simulink model "ccu_form"  (R2019b)
settings: Solver=FixedStepDiscrete  StartTime=0.0  StopTime=10.0  FixedStep=0.0005  RelTol=1e-3
undefined symbols (not defined in the file): CubeAndKeil, DiscIntNeverNeededParam, Ggg2
libraries: simulink x6, GPIO_Lib x5, ADC_Lib x2, TIMERS_Lib x2, USART_Lib x2, STM32_Config_Lib x1
settings Model: Creator=Guest  LastModifiedBy=Dmitry
settings OptimizationCC: DefaultParameterBehavior=Inlined  OptimizeBlockIOStorage=off  BufferReuse=off  GlobalBufferReuse=off  ExpressionFolding=off  EnableMemcpy=off  PassReuseOutputArgsAs=Individual arguments  LocalBlockOutputs=off  ZeroExternalMemoryAtStartup=off  ZeroInternalMemoryAtStartup=off  OptimizeDataStoreBuffers=off  BusAssignmentInplaceUpdate=off  OptimizationLevel=level0  OptimizationCustomize=off  EfficientTunableParamExpr=on
settings DebuggingCC: MultiTaskDSMMsg=none  ParameterOverflowMsg=none  ParameterTunabilityLossMsg=error
settings HardwareCC: ProdBitPerPointer=32  ProdBitPerSizeT=32  ProdBitPerPtrDiffT=32  ProdLargestAtomicInteger=Long  ProdWordSize=32  ProdHWDeviceType=STM32CortexM
settings SFSimCC: MATLABDynamicMemAlloc=off
settings RTWCC: Description=stm32 (Embedded Target)  SystemTargetFile=stm32.tlc  TemplateMakefile=stm32.tmf  GenerateReport=on  IncludeHyperlinkInReport=on  GenerateTraceInfo=on  GenerateTraceReport=on  GenerateTraceReportSl=on  GenerateTraceReportSf=on  GenerateTraceReportEml=on
settings CodeAppCC: ForceParamTrailComments=on  IgnoreCustomStorageClasses=off  MaxIdLength=64  OperatorAnnotations=on  SimulinkDataObjDesc=on  SFDataObjDesc=on  CustomSymbolStrType=$N$R$M
settings STFCustomTargetCC: TargetLangStandard=C99 (ISO)  CodeReplacementLibrary=ARM CMSIS SIN COS  MultiwordLength=256  ParMdlRefBuildCompliant=on  IncludeMdlTerminateFcn=off  CombineOutputUpdateFcns=on  ERTCustomFileBanners=on  SupportContinuousTime=off  SupportNonInlinedSFcns=off  RemoveResetFunc=on  MATLABClassNameForMDSCustomization=Simulink.SoftwareTarget.ERTCustomization  SystemTargetFile=stm32.tlc
settings ERTTargetCC: TargetLangStandard=C99 (ISO)  CodeReplacementLibrary=ARM CMSIS SIN COS  CompOptLevelCompliant=off  ConcurrentExecutionCompliant=off  IncludeMdlTerminateFcn=off  ModelStepFunctionPrototypeControlCompliant=off  CPPClassGenCompliant=off  UseToolchainInfoCompliant=off  ExtModeStaticAllocSize=256  ExtModeMexFile=ext_serial_win32_comm  ExtModeMexArgs=0,1,115200,10  InlinedParameterPlacement=NonHierarchical  ERTSrcFileBannerTemplate=sourceFileTemplate.cgt  ERTHdrFileBannerTemplate=sourceFileTemplate.cgt  ERTDataSrcFileTemplate=sourceFileTemplate.cgt  ERTDataHdrFileTemplate=sourceFileTemplate.cgt  ERTCustomFileTemplate=customRoutineProcess.tlc

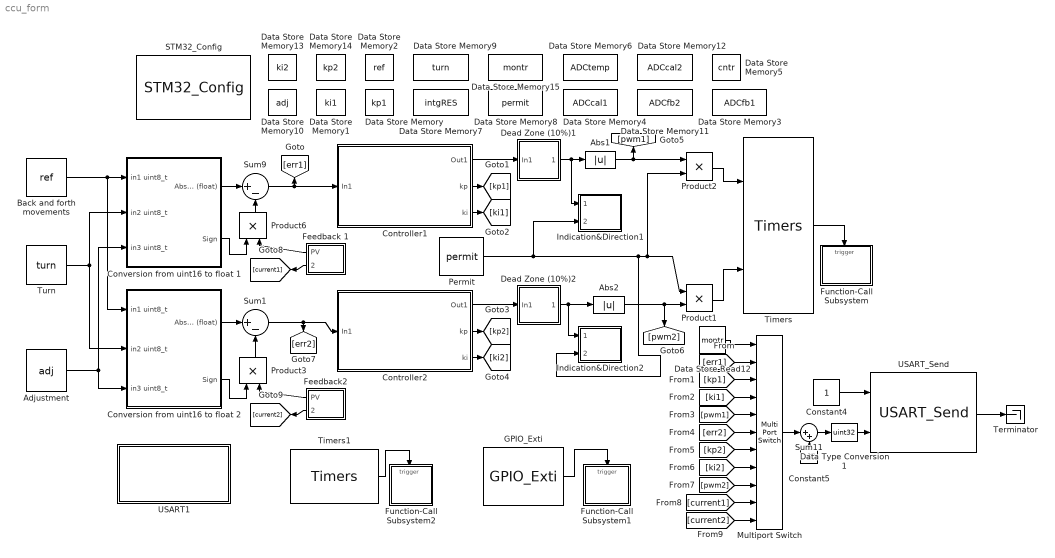
== system ccu_form ==
  Abs1 : Abs
  Abs2 : Abs
  Adjustment : DataStoreRead  DataStoreName=adj  DataStoreElements=adj
      mask Display: image('E:\diplom\matlab\handle.png','center')
  Back and forth movements : DataStoreRead  DataStoreName=ref  DataStoreElements=ref
      mask Display: image('E:\diplom\matlab\joystick_fb.png','center')
  Constant4 : Constant
  Constant5 : Constant  Value=100  OutDataTypeStr=uint8
  Controller1 : Subsystem
      mask Display: image('E:\diplom\matlab\pi.png','center')
  Controller2 : Subsystem
      mask Display: image('E:\diplom\matlab\pi.png','center')
  Conversion from uint16 to float 1 : Subsystem
  Conversion from uint16 to float 2 : Subsystem
  Data Store Memory : DataStoreMemory  DataStoreName=kp1  ReadBeforeWriteMsg=warning  WriteAfterWriteMsg=warning  WriteAfterReadMsg=warning  ShowAdditionalParam=off  OutDataTypeStr=uint8
  Data Store Memory1 : DataStoreMemory  DataStoreName=ki1  ReadBeforeWriteMsg=warning  WriteAfterWriteMsg=warning  WriteAfterReadMsg=warning  ShowAdditionalParam=off  OutDataTypeStr=uint8
  Data Store Memory10 : DataStoreMemory  DataStoreName=adj  ReadBeforeWriteMsg=warning  WriteAfterWriteMsg=warning  WriteAfterReadMsg=warning  ShowAdditionalParam=off  OutDataTypeStr=uint8
  Data Store Memory11 : DataStoreMemory  DataStoreName=ADCfb2  ReadBeforeWriteMsg=warning  WriteAfterWriteMsg=warning  WriteAfterReadMsg=warning  ShowAdditionalParam=off  OutDataTypeStr=uint16
  Data Store Memory12 : DataStoreMemory  DataStoreName=ADCcal2  ReadBeforeWriteMsg=warning  WriteAfterWriteMsg=warning  WriteAfterReadMsg=warning  ShowAdditionalParam=off  OutDataTypeStr=uint16
  Data Store Memory13 : DataStoreMemory  DataStoreName=ki2  ReadBeforeWriteMsg=warning  WriteAfterWriteMsg=warning  WriteAfterReadMsg=warning  ShowAdditionalParam=off  OutDataTypeStr=uint8
  Data Store Memory14 : DataStoreMemory  DataStoreName=kp2  ReadBeforeWriteMsg=warning  WriteAfterWriteMsg=warning  WriteAfterReadMsg=warning  ShowAdditionalParam=off  OutDataTypeStr=uint8
  Data Store Memory15 : DataStoreMemory  DataStoreName=montr  ReadBeforeWriteMsg=warning  WriteAfterWriteMsg=warning  WriteAfterReadMsg=warning  ShowAdditionalParam=off  OutDataTypeStr=uint8
  Data Store Memory2 : DataStoreMemory  DataStoreName=ref  ReadBeforeWriteMsg=warning  WriteAfterWriteMsg=warning  WriteAfterReadMsg=warning  ShowAdditionalParam=off  OutDataTypeStr=uint8
  Data Store Memory3 : DataStoreMemory  DataStoreName=ADCfb1  ReadBeforeWriteMsg=warning  WriteAfterWriteMsg=warning  WriteAfterReadMsg=warning  ShowAdditionalParam=off  OutDataTypeStr=uint16
  Data Store Memory4 : DataStoreMemory  DataStoreName=ADCcal1  ReadBeforeWriteMsg=warning  WriteAfterWriteMsg=warning  WriteAfterReadMsg=warning  ShowAdditionalParam=off  OutDataTypeStr=uint16
  Data Store Memory5 : DataStoreMemory  DataStoreName=cntr  ReadBeforeWriteMsg=warning  WriteAfterWriteMsg=warning  WriteAfterReadMsg=warning  ShowAdditionalParam=off  OutDataTypeStr=uint16
  Data Store Memory6 : DataStoreMemory  DataStoreName=ADCtemp  ReadBeforeWriteMsg=warning  WriteAfterWriteMsg=warning  WriteAfterReadMsg=warning  ShowAdditionalParam=off  OutDataTypeStr=uint32
  Data Store Memory7 : DataStoreMemory  DataStoreName=intgRES  ReadBeforeWriteMsg=warning  WriteAfterWriteMsg=warning  WriteAfterReadMsg=warning  ShowAdditionalParam=off  OutDataTypeStr=uint8
  Data Store Memory8 : DataStoreMemory  DataStoreName=permit  ReadBeforeWriteMsg=warning  WriteAfterWriteMsg=warning  WriteAfterReadMsg=warning  ShowAdditionalParam=off  OutDataTypeStr=uint8
  Data Store Memory9 : DataStoreMemory  DataStoreName=turn  ReadBeforeWriteMsg=warning  WriteAfterWriteMsg=warning  WriteAfterReadMsg=warning  ShowAdditionalParam=off  OutDataTypeStr=uint8
  Data Store Read12 : DataStoreRead  DataStoreName=montr  DataStoreElements=montr
  Data Type Conversion1 : DataTypeConversion  OutDataTypeStr=uint32
  Dead Zone (10%)1 : Subsystem
      mask Display:
      | plot([0.01 1 1.01 3 3.01 4.01],[-1.00001 -0.5 0.00001 0 0.5 1.01])
      | plot([0.0001 1.0001 1.0001 3.0001 3.0001 4.00001],[-1.0001 -0.50001 0.0001 0.0001 0.5001 1.0001])
      | plot([0.0002 1.0002 1.001 3.001 3.001 4.0001],[-1.0005 -0.50005 0.0005 0.0005 0.5005 1.0005])
      | plot([2 2],[-1 1])
      | plot([0 4],[0 0])
  Dead Zone (10%)2 : Subsystem
      mask Display:
      | plot([0.01 1 1.01 3 3.01 4.01],[-1.00001 -0.5 0.00001 0 0.5 1.01])
      | plot([0.0001 1.0001 1.0001 3.0001 3.0001 4.00001],[-1.0001 -0.50001 0.0001 0.0001 0.5001 1.0001])
      | plot([0.0002 1.0002 1.001 3.001 3.001 4.0001],[-1.0005 -0.50005 0.0005 0.0005 0.5005 1.0005])
      | plot([2 2],[-1 1])
      | plot([0 4],[0 0])
  Feedback 1 : Subsystem
  Feedback2 : Subsystem
  Function-Call Subsystem : Subsystem  TreatAsAtomicUnit=on
  Function-Call Subsystem1 : Subsystem  TreatAsAtomicUnit=on
  Function-Call Subsystem2 : Subsystem  TreatAsAtomicUnit=on
  GPIO_Exti : GPIO_Lib/GPIO_Exti  Port_name=GPIOA  Pin_0=off  Pin_1=off  Pin_2=off  Pin_3=off  Pin_4=on  Pin_5=off  Pin_6=off  Pin_7=off  Pin_8=off  Pin_9=off  Pin_10=off  Pin_11=off  Pin_12=off  Pin_13=off  Pin_14=off  Pin_15=off  PinList=GPIOA4
      settings: SourceProductName=Target Support Package - STM32 Adapter
  Indication&Direction1 : Subsystem
  Indication&Direction2 : Subsystem
  Multiport Switch : MultiPortSwitch  Inputs=10  OutDataTypeStr=uint8
  Permit : DataStoreRead  DataStoreName=permit  DataStoreElements=permit
      mask Display: image('E:\diplom\matlab\switch.png','center')
  Product1 : Product
  Product2 : Product
  Product3 : Product  OutDataTypeStr=double
  Product6 : Product  OutDataTypeStr=double
  STM32_Config : STM32_Config_Lib/STM32_Config  Priority=0  Project_Path=.\..\CubeAndKeil\Ggg2\  Config_File=Ggg2.ioc  MCU_Name=STM32F401CCUx
      settings: SourceProductName=Target Support Package - STM32 Adapter
  Sum1 : Sum  Inputs=|+-  AccumDataTypeStr=double  OutDataTypeStr=double
  Sum11 : Sum  Inputs=|++  AccumDataTypeStr=double  OutDataTypeStr=double
  Sum9 : Sum  Inputs=|+-  AccumDataTypeStr=double  OutDataTypeStr=double
  Terminator : Terminator
  Timers : TIMERS_Lib/Timers  currentTIM=TIM1  TIM_Name=TIM1  sysUsingTimer=off  TIM_APBClock=84000000  TIM_Set_Clk=off  TIM_Prescaler=0  TIM_Clock=84000000.00  Variable_frequency=off  TIM_Set_OutFreq=off  TIM_ARR=4201  Output_frequency=19995.24  Repetition_counter=0  TIM_Mode=Center_Aligned_3  TIM_DMA=none  TIM_IRQ=on  TIM_IRQ_ONLY=off  TIM_UP=off  TIM_TRG=off  TIM_COM=off  TIM_BRK=off  NbTIM=2  CH1_enable=on  CH1N_enable=on  CH1_type=Output_PWM  CH1_DMA=off  CH1_int=off  CH1_edge=Rising  CH1_div=1  CH1_variable_duty=on  CH1_set_pulse=off  CH1_output_duty=49.99  CH1_pulse=2100  CH2_enable=on  CH2N_enable=off  CH2_type=Output_Comp  CH2_DMA=off  CH2_int=on  CH2_edge=Rising  CH2_div=1  CH2_variable_duty=off  CH2_set_pulse=off  CH2_output_duty=0.00  CH2_pulse=0  CH3_enable=on  CH3N_enable=off  CH3_type=Output_PWM  CH3_DMA=off  CH3_int=off  CH3_edge=Rising  CH3_div=1  CH3_variable_duty=on  CH3_set_pulse=off  CH3_output_duty=49.99  CH3_pulse=2100  CH4_enable=off  CH4N_enable=off  CH4_type=Unknown  CH4_DMA=off  CH4_int=off  CH4_edge=Rising  CH4_div=1  CH4_variable_duty=off  CH4_set_pulse=off  CH4_output_duty=0.00  CH4_pulse=0
      settings: SourceProductName=Target Support Package - STM32 Adapter
  Timers1 : TIMERS_Lib/Timers  currentTIM=TIM2  TIM_Name=TIM2  sysUsingTimer=off  TIM_APBClock=84000000  TIM_Set_Clk=off  TIM_Prescaler=839  TIM_Clock=100000.00  Variable_frequency=off  TIM_Set_OutFreq=off  TIM_ARR=51  Output_frequency=1960.78  Repetition_counter=0  TIM_Mode=Up  TIM_DMA=none  TIM_IRQ=on  TIM_IRQ_ONLY=off  TIM_UP=on  TIM_TRG=off  TIM_COM=off  TIM_BRK=off  NbTIM=2  CH1_enable=on  CH1N_enable=off  CH1_type=Output_Comp  CH1_DMA=off  CH1_int=off  CH1_edge=Rising  CH1_div=1  CH1_variable_duty=off  CH1_set_pulse=off  CH1_output_duty=0.00  CH1_pulse=0  CH2_enable=off  CH2N_enable=off  CH2_type=Unknown  CH2_DMA=off  CH2_int=off  CH2_edge=Rising  CH2_div=1  CH2_variable_duty=off  CH2_set_pulse=off  CH2_output_duty=0.00  CH2_pulse=0  CH3_enable=off  CH3N_enable=off  CH3_type=Unknown  CH3_DMA=off  CH3_int=off  CH3_edge=Rising  CH3_div=1  CH3_variable_duty=off  CH3_set_pulse=off  CH3_output_duty=0.00  CH3_pulse=0  CH4_enable=off  CH4N_enable=off  CH4_type=Unknown  CH4_DMA=off  CH4_int=off  CH4_edge=Rising  CH4_div=1  CH4_variable_duty=off  CH4_set_pulse=off  CH4_output_duty=0.00  CH4_pulse=0
      settings: SourceProductName=Target Support Package - STM32 Adapter
  Turn : DataStoreRead  DataStoreName=turn  DataStoreElements=turn
      mask Display: image('E:\diplom\matlab\joystick_TURN.png','center')
  USART1 : Subsystem
      mask Display: disp('USART1 Recieve')
  USART_Send : USART_Lib/USART_Send  USART_name=USART2  Buff_size=512  nbUsart=2  usartMode=Asynchronous  usartDma_Rx=off  usartDma_Tx=off  usartIt=on
      settings: SourceProductName=Target Support Package - STM32 Adapter
  wires:
  Timers/1 -> Function-Call Subsystem/Trigger
  GPIO_Exti/1 -> Function-Call Subsystem1/Trigger
  Timers1/1 -> Function-Call Subsystem2/Trigger
  Product2/1 -> Timers/1
  Product6/1 -> Sum9/2
  Abs1/1 -> Product2/1, [pwm1]
  Sum9/1 -> [err1], Controller1/1(In1)
  Dead Zone (10%)1/1(Out1) -> Abs1/1, Indication&Direction1/1(direction)
  Controller1/1(Out1) -> Dead Zone (10%)1/1(In1)
  Feedback 1/1(PV) -> Product6/2
  Conversion from uint16 to float 1/1("Absolute units SP (float) ") -> Sum9/1
  Conversion from uint16 to float 1/2(Sign) -> Product6/1
  Conversion from uint16 to float 2/2(Sign) -> Product3/1
  Conversion from uint16 to float 2/1("Absolute units SP (float) ") -> Sum1/1
  Feedback2/1(PV) -> Product3/2
  Controller2/1(Out1) -> Dead Zone (10%)2/1(In1)
  Dead Zone (10%)2/1(Out1) -> Abs2/1, Indication&Direction2/1(direction)
  Sum1/1 -> Controller2/1(In1), [err2]
  Abs2/1 -> Product1/2, [pwm2]
  Product3/1 -> Sum1/2
  Product1/1 -> Timers/2
  Turn/1 -> Conversion from uint16 to float 2/2(in2 uint8_t), Conversion from uint16 to float 1/2(in2 uint8_t)
  Adjustment/1 -> Conversion from uint16 to float 2/3(in3 uint8_t), Conversion from uint16 to float 1/3(in3 uint8_t)
  Controller1/2(kp) -> [kp1]
  Controller1/3(ki) -> [ki1]
  Controller2/3(ki) -> [ki2]
  Controller2/2(kp) -> [kp2]
  Feedback 1/2(current) -> [current1]
  Feedback2/2(current) -> [current2]
  Back and forth movements/1 -> Conversion from uint16 to float 1/1(in1 uint8_t), Conversion from uint16 to float 2/1(in1 uint8_t)
  Permit/1 -> Product2/2, Product1/1, Indication&Direction2/2(indication), Indication&Direction1/2(indication)
  [err1] -> Multiport Switch/2
  [current1] -> Multiport Switch/10
  Constant5/1 -> Sum11/2
  [pwm2] -> Multiport Switch/9
  Multiport Switch/1 -> Sum11/1
  Data Type Conversion1/1 -> USART_Send/2
  [err2] -> Multiport Switch/6
  Constant4/1 -> USART_Send/1
  USART_Send/1 -> Terminator/1
  [kp1] -> Multiport Switch/3
  [ki1] -> Multiport Switch/4
  Sum11/1 -> Data Type Conversion1/1
  [pwm1] -> Multiport Switch/5
  [ki2] -> Multiport Switch/8
  [kp2] -> Multiport Switch/7
  Data Store Read12/1 -> Multiport Switch/1
  [current2] -> Multiport Switch/11

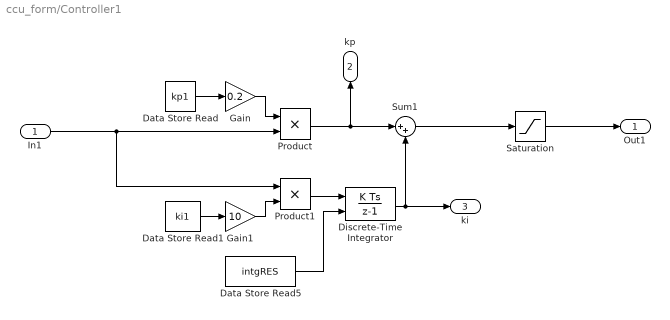
== system ccu_form/Controller1 ==
  In1 : Inport
  Data Store Read : DataStoreRead  DataStoreName=kp1  DataStoreElements=kp1
  Data Store Read1 : DataStoreRead  DataStoreName=ki1  DataStoreElements=ki1
  Data Store Read5 : DataStoreRead  DataStoreName=intgRES  DataStoreElements=intgRES
  Discrete-Time Integrator : DiscreteIntegrator  ExternalReset=level  SampleTime=-1  LimitOutput=on  UpperSaturationLimit=100  LowerSaturationLimit=-100  ICPrevOutput=DiscIntNeverNeededParam  ICPrevScaledInput=DiscIntNeverNeededParam
  Gain : Gain  Gain=0.2  OutDataTypeStr=single
  Gain1 : Gain  Gain=10  OutDataTypeStr=single
  Product : Product  OutDataTypeStr=double
  Product1 : Product  OutDataTypeStr=double
  Saturation : Saturate  UpperLimit=100  LowerLimit=-100
  Sum1 : Sum  Inputs=|++
  Out1 : Outport
  kp : Outport  Port=2
  ki : Outport  Port=3
  wires:
  Data Store Read1/1 -> Gain1/1
  In1/1 -> Product1/1, Product/2
  Product1/1 -> Discrete-Time Integrator/1
  Product/1 -> kp/1, Sum1/1
  Data Store Read/1 -> Gain/1
  Sum1/1 -> Saturation/1
  Data Store Read5/1 -> Discrete-Time Integrator/2
  Discrete-Time Integrator/1 -> Sum1/2, ki/1
  Gain/1 -> Product/1
  Gain1/1 -> Product1/2
  Saturation/1 -> Out1/1

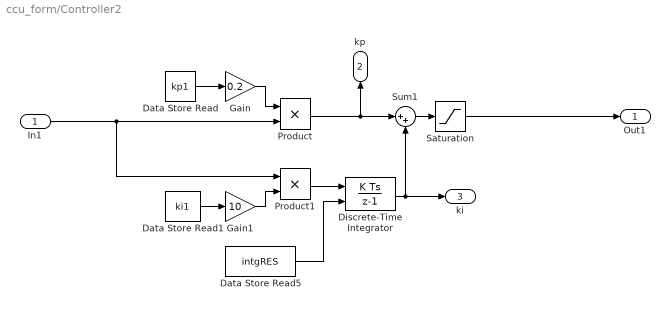
== system ccu_form/Controller2 ==
  In1 : Inport
  Data Store Read : DataStoreRead  DataStoreName=kp1  DataStoreElements=kp1
  Data Store Read1 : DataStoreRead  DataStoreName=ki1  DataStoreElements=ki1
  Data Store Read5 : DataStoreRead  DataStoreName=intgRES  DataStoreElements=intgRES
  Discrete-Time Integrator : DiscreteIntegrator  ExternalReset=level  SampleTime=-1  LimitOutput=on  UpperSaturationLimit=100  LowerSaturationLimit=-100  ICPrevOutput=DiscIntNeverNeededParam  ICPrevScaledInput=DiscIntNeverNeededParam
  Gain : Gain  Gain=0.2  OutDataTypeStr=single
  Gain1 : Gain  Gain=10  OutDataTypeStr=single
  Product : Product  OutDataTypeStr=double
  Product1 : Product  OutDataTypeStr=double
  Saturation : Saturate  UpperLimit=100  LowerLimit=-100
  Sum1 : Sum  Inputs=|++
  Out1 : Outport
  kp : Outport  Port=2
  ki : Outport  Port=3
  wires:
  Saturation/1 -> Out1/1
  Gain1/1 -> Product1/2
  Gain/1 -> Product/1
  Discrete-Time Integrator/1 -> ki/1, Sum1/2
  Data Store Read5/1 -> Discrete-Time Integrator/2
  Sum1/1 -> Saturation/1
  Data Store Read/1 -> Gain/1
  Product/1 -> kp/1, Sum1/1
  Product1/1 -> Discrete-Time Integrator/1
  In1/1 -> Product/2, Product1/1
  Data Store Read1/1 -> Gain1/1

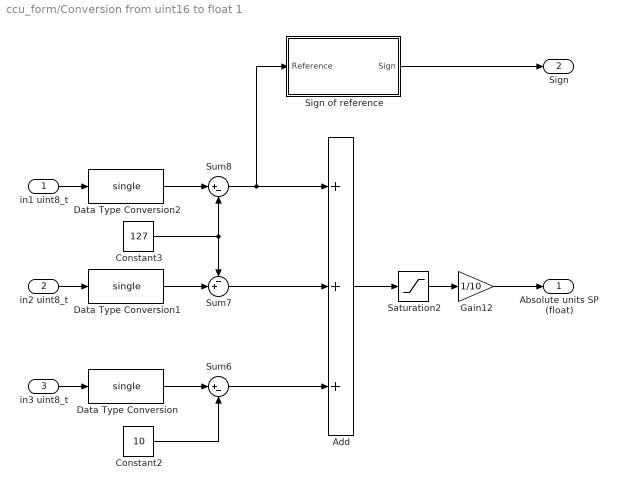
== system ccu_form/Conversion from uint16 to float 1 ==
  in1 uint8_t : Inport
  in2 uint8_t : Inport  Port=2
  in3 uint8_t : Inport  Port=3
  Add : Sum  Inputs=3
  Constant2 : Constant  Value=10  OutDataTypeStr=single
  Constant3 : Constant  Value=127  OutDataTypeStr=single
  Data Type Conversion : DataTypeConversion  OutDataTypeStr=single
  Data Type Conversion1 : DataTypeConversion  OutDataTypeStr=single
  Data Type Conversion2 : DataTypeConversion  OutDataTypeStr=single
  Gain12 : Gain  Gain=1/10  OutDataTypeStr=double
  Saturation2 : Saturate  UpperLimit=127  LowerLimit=-127
  Sign of reference : Subsystem
  Sum6 : Sum  Inputs=|+-  AccumDataTypeStr=double  OutDataTypeStr=double
  Sum7 : Sum  Inputs=-+|  AccumDataTypeStr=double  OutDataTypeStr=double
  Sum8 : Sum  Inputs=|+-  AccumDataTypeStr=double  OutDataTypeStr=double
  "Absolute units SP (float) " : Outport
  Sign : Outport  Port=2
  wires:
  in2 uint8_t/1 -> Data Type Conversion1/1
  Sum8/1 -> Sign of reference/1(Reference), Add/1
  Data Type Conversion1/1 -> Sum7/2
  Constant3/1 -> Sum7/1, Sum8/2
  Add/1 -> Saturation2/1
  Saturation2/1 -> Gain12/1
  Sum6/1 -> Add/3
  in1 uint8_t/1 -> Data Type Conversion2/1
  Gain12/1 -> "Absolute units SP (float) "/1
  Data Type Conversion2/1 -> Sum8/1
  Data Type Conversion/1 -> Sum6/1
  Constant2/1 -> Sum6/2
  Sum7/1 -> Add/2
  in3 uint8_t/1 -> Data Type Conversion/1
  Sign of reference/1(Sign) -> Sign/1

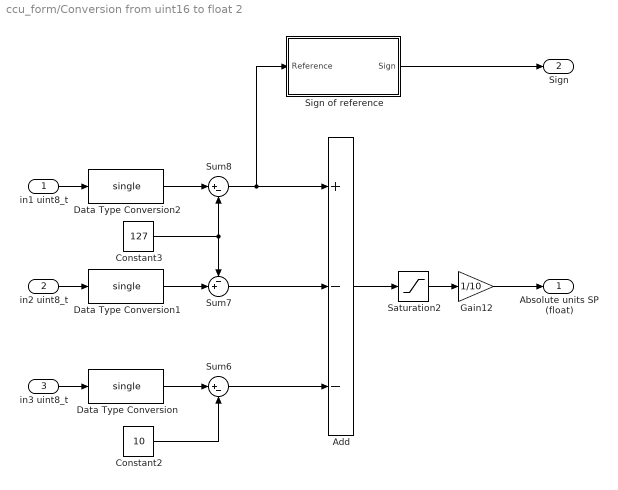
== system ccu_form/Conversion from uint16 to float 2 ==
  in1 uint8_t : Inport
  in2 uint8_t : Inport  Port=2
  in3 uint8_t : Inport  Port=3
  Add : Sum  Inputs=+--
  Constant2 : Constant  Value=10  OutDataTypeStr=single
  Constant3 : Constant  Value=127  OutDataTypeStr=single
  Data Type Conversion : DataTypeConversion  OutDataTypeStr=single
  Data Type Conversion1 : DataTypeConversion  OutDataTypeStr=single
  Data Type Conversion2 : DataTypeConversion  OutDataTypeStr=single
  Gain12 : Gain  Gain=1/10  OutDataTypeStr=double
  Saturation2 : Saturate  UpperLimit=127  LowerLimit=-127
  Sign of reference : Subsystem
  Sum6 : Sum  Inputs=|+-  AccumDataTypeStr=double  OutDataTypeStr=double
  Sum7 : Sum  Inputs=-+|  AccumDataTypeStr=double  OutDataTypeStr=double
  Sum8 : Sum  Inputs=|+-  AccumDataTypeStr=double  OutDataTypeStr=double
  "Absolute units SP (float) " : Outport
  Sign : Outport  Port=2
  wires:
  Sign of reference/1(Sign) -> Sign/1
  in3 uint8_t/1 -> Data Type Conversion/1
  Sum7/1 -> Add/2
  Constant2/1 -> Sum6/2
  Data Type Conversion/1 -> Sum6/1
  Data Type Conversion2/1 -> Sum8/1
  Gain12/1 -> "Absolute units SP (float) "/1
  in1 uint8_t/1 -> Data Type Conversion2/1
  Sum6/1 -> Add/3
  Saturation2/1 -> Gain12/1
  Add/1 -> Saturation2/1
  Constant3/1 -> Sum8/2, Sum7/1
  Data Type Conversion1/1 -> Sum7/2
  Sum8/1 -> Add/1, Sign of reference/1(Reference)
  in2 uint8_t/1 -> Data Type Conversion1/1

== system ccu_form/Dead Zone (10%)1 ==
  In1 : Inport
  Abs : Abs
  Constant : Constant  Value=0
  Switch : Switch  Criteria=u2 > Threshold  Threshold=10
  Out1 : Outport
  wires:
  In1/1 -> Switch/1, Abs/1
  Abs/1 -> Switch/2
  Constant/1 -> Switch/3
  Switch/1 -> Out1/1

== system ccu_form/Dead Zone (10%)2 ==
  In1 : Inport
  Abs : Abs
  Constant : Constant  Value=0
  Switch : Switch  Criteria=u2 > Threshold  Threshold=10
  Out1 : Outport
  wires:
  Switch/1 -> Out1/1
  Constant/1 -> Switch/3
  Abs/1 -> Switch/2
  In1/1 -> Abs/1, Switch/1

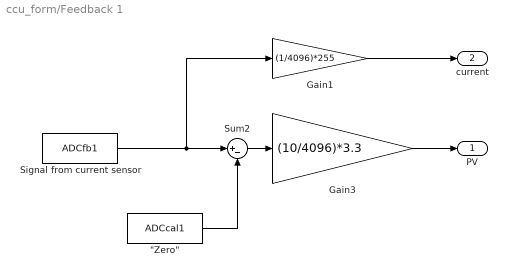
== system ccu_form/Feedback 1 ==
  "\"Zero\"" : DataStoreRead  DataStoreName=ADCcal1  DataStoreElements=ADCcal1
  Gain1 : Gain  Gain=(1/4096)*255  OutDataTypeStr=double
  Gain3 : Gain  Gain=(10/4096)*3.3  OutDataTypeStr=double
  Signal from current sensor : DataStoreRead  DataStoreName=ADCfb1  DataStoreElements=ADCfb1
  Sum2 : Sum  Inputs=|+-  AccumDataTypeStr=double  OutDataTypeStr=double
  PV : Outport
  current : Outport  Port=2
  wires:
  "\"Zero\""/1 -> Sum2/2
  Gain3/1 -> PV/1
  Signal from current sensor/1 -> Gain1/1, Sum2/1
  Sum2/1 -> Gain3/1
  Gain1/1 -> current/1

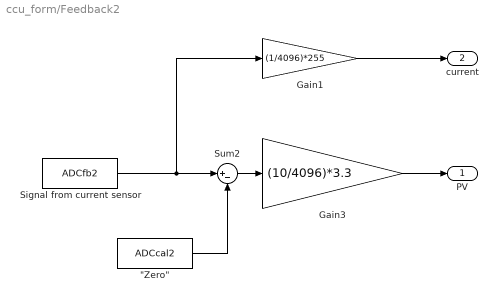
== system ccu_form/Feedback2 ==
  "\"Zero\"" : DataStoreRead  DataStoreName=ADCcal2  DataStoreElements=ADCcal2
  Gain1 : Gain  Gain=(1/4096)*255  OutDataTypeStr=double
  Gain3 : Gain  Gain=(10/4096)*3.3  OutDataTypeStr=double
  Signal from current sensor : DataStoreRead  DataStoreName=ADCfb2  DataStoreElements=ADCfb2
  Sum2 : Sum  Inputs=|+-  AccumDataTypeStr=double  OutDataTypeStr=double
  PV : Outport
  current : Outport  Port=2
  wires:
  Sum2/1 -> Gain3/1
  Gain3/1 -> PV/1
  "\"Zero\""/1 -> Sum2/2
  Signal from current sensor/1 -> Gain1/1, Sum2/1
  Gain1/1 -> current/1

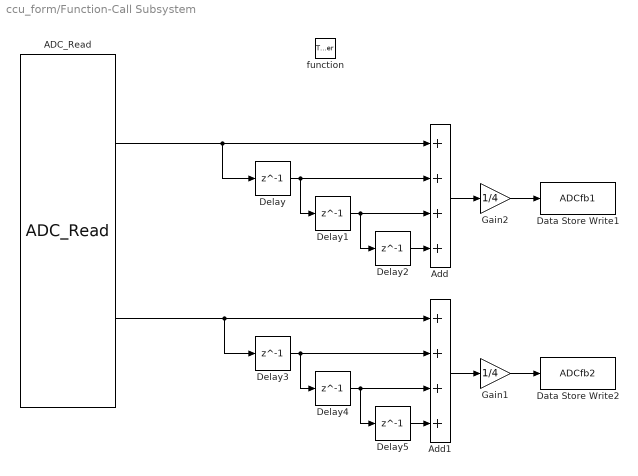
== system ccu_form/Function-Call Subsystem ==
  function : TriggerPort  TriggerType=function-call  VariantControl=Variant
  ADC_Read : ADC_Lib/ADC_Read  ADC_Name=ADC1  ADC_Ch0=on  ADC_Ch1=on  ADC_Ch2=off  ADC_Ch3=off  ADC_Ch4=off  ADC_Ch5=on  ADC_Ch6=off  ADC_Ch7=off  ADC_Ch8=off  ADC_Ch9=off  ADC_Ch10=off  ADC_Ch11=off  ADC_Ch12=off  ADC_Ch13=off  ADC_Ch14=off  ADC_Ch15=off  ADC_Ch16=off  ADC_Ch17=off  ADC_Ch18=off  RgRk1=on  RgRk2=on  RgRk3=off  RgRk4=off  RgRk1_Ch=Ch0_r1  RgRk2_Ch=Ch1_r2  RgRk3_Ch=off  RgRk4_Ch=off  RgRk5=off  RgRk6=off  RgRk7=off  RgRk8=off  RgRk5_Ch=off  RgRk6_Ch=off  RgRk7_Ch=off  RgRk8_Ch=off  RgRk9=off  RgRk10=off  RgRk11=off  RgRk12=off  RgRk9_Ch=off  RgRk10_Ch=off  RgRk11_Ch=off  RgRk12_Ch=off  RgRk13=off  RgRk14=off  RgRk15=off  RgRk16=off  RgRk13_Ch=off  RgRk14_Ch=off  RgRk15_Ch=off  RgRk16_Ch=off  InjRk1=off  InjRk2=off  InjRk3=off  InjRk4=off  InjRk1_Ch=off  InjRk2_Ch=off  InjRk3_Ch=off  InjRk4_Ch=off  ADC_Trig=Not used  ADC_TrigEdge=Not used  DmaReq=off  DMA_Buffer=0  ItReq=off  AWD_Mode=NOT_USED  AWD_Ch=0  AWD_HThres=0  AWD_LThres=0  AWD_En_Int=off  AWD2_HThres=0  AWD2_LThres=0  AWD2_En_Int=off  AWD3_HThres=0  AWD3_LThres=0  AWD3_En_Int=off  EOC_SEQ=off  EOC_IT=off  JEOC_IT=off  AWD_IT=off  OVR_IT=off  CpltTrans=off  HalfTrans=off  ADC_RegNb=2  ADC_RegCh0=on  ADC_RegCh1=on  ADC_RegCh2=off  ADC_RegCh3=off  ADC_RegCh4=off  ADC_RegCh5=on  ADC_RegCh6=off  ADC_RegCh7=off  ADC_RegCh8=off  ADC_RegCh9=off  ADC_RegCh10=off  ADC_RegCh11=off  ADC_RegCh12=off  ADC_RegCh13=off  ADC_RegCh14=off  ADC_RegCh15=off  ADC_RegCh16=off  ADC_RegCh17=off  ADC_RegCh18=off  ADC_InjNb=2  ADC_InjCh0=off  ADC_InjCh1=on  ADC_InjCh2=off  ADC_InjCh3=off  ADC_InjCh4=off  ADC_InjCh5=on  ADC_InjCh6=on  ADC_InjCh7=off  ADC_InjCh8=off  ADC_InjCh9=off  ADC_InjCh10=off  ADC_InjCh11=off  ADC_InjCh12=off  ADC_InjCh13=off  ADC_InjCh14=off  ADC_InjCh15=off  ADC_InjCh16=off  ADC_InjCh17=off  ADC_InjCh18=off  ADC_RegRank0=1  ADC_RegRank1=2  ADC_RegRank2=0  ADC_RegRank3=0  ADC_RegRank4=0  ADC_RegRank5=2  ADC_RegRank6=0  ADC_RegRank7=0  ADC_RegRank8=0  ADC_RegRank9=0  ADC_RegRank10=0  ADC_RegRank11=0  ADC_RegRank12=0  ADC_RegRank13=0  ADC_RegRank14=0  ADC_RegRank15=0  ADC_RegRank16=0  ADC_RegRank17=0  ADC_RegRank18=0  ADC_InjRank0=0  ADC_InjRank1=0  ADC_InjRank2=0  ADC_InjRank3=0  ADC_InjRank4=0  ADC_InjRank5=0  ADC_InjRank6=0  ADC_InjRank7=0  ADC_InjRank8=0  ADC_InjRank9=0  ADC_InjRank10=0  ADC_InjRank11=0  ADC_InjRank12=0  ADC_InjRank13=0  ADC_InjRank14=0  ADC_InjRank15=0  ADC_InjRank16=0  ADC_InjRank17=0  ADC_InjRank18=0  NbADC=1  CurrentADC=ADC1
      settings: SourceProductName=Target Support Package - STM32 Adapter
  Add : Sum  Inputs=++++
  Add1 : Sum  Inputs=++++
  Data Store Write1 : DataStoreWrite  DataStoreName=ADCfb1  DataStoreElements=ADCfb1
  Data Store Write2 : DataStoreWrite  DataStoreName=ADCfb2  DataStoreElements=ADCfb2
  Delay{,1..5} (6 alike) : Delay  DelayLength=1  InitialCondition=0
  Gain1 : Gain  Gain=1/4  OutDataTypeStr=uint16
  Gain2 : Gain  Gain=1/4  OutDataTypeStr=uint16
  wires:
  Delay/1 -> Add/2, Delay1/1
  Delay1/1 -> Delay2/1, Add/3
  Add/1 -> Gain2/1
  ADC_Read/1 -> Delay/1, Add/1
  Delay2/1 -> Add/4
  Gain2/1 -> Data Store Write1/1
  Gain1/1 -> Data Store Write2/1
  Delay5/1 -> Add1/4
  ADC_Read/2 -> Delay3/1, Add1/1
  Delay4/1 -> Add1/3, Delay5/1
  Delay3/1 -> Delay4/1, Add1/2
  Add1/1 -> Gain1/1

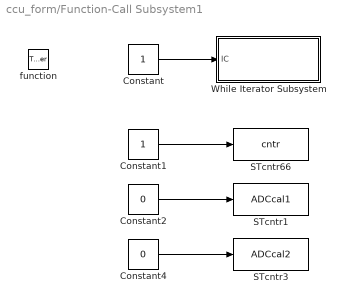
== system ccu_form/Function-Call Subsystem1 ==
  function : TriggerPort  TriggerType=function-call  VariantControl=Variant
  Constant : Constant  OutDataTypeStr=boolean
  Constant1 : Constant  OutDataTypeStr=uint16
  Constant2 : Constant  Value=0  OutDataTypeStr=uint16
  Constant4 : Constant  Value=0  OutDataTypeStr=uint16
  STcntr1 : DataStoreWrite  DataStoreName=ADCcal1  DataStoreElements=ADCcal1
  STcntr3 : DataStoreWrite  DataStoreName=ADCcal2  DataStoreElements=ADCcal2
  STcntr66 : DataStoreWrite  DataStoreName=cntr  DataStoreElements=cntr
  While Iterator Subsystem : Subsystem  TreatAsAtomicUnit=on
  wires:
  Constant/1 -> While Iterator Subsystem/1(IC)
  Constant1/1 -> STcntr66/1
  Constant2/1 -> STcntr1/1
  Constant4/1 -> STcntr3/1

== system ccu_form/Function-Call Subsystem2 ==
  function : TriggerPort  TriggerType=function-call  VariantControl=Variant
  AddQQ : Sum
  Constant543 : Constant  OutDataTypeStr=uint8
  STcntr54 : DataStoreRead  DataStoreName=cntr  DataStoreElements=cntr
  STcntr67 : DataStoreWrite  DataStoreName=cntr  DataStoreElements=cntr
  wires:
  STcntr54/1 -> AddQQ/2
  AddQQ/1 -> STcntr67/1
  Constant543/1 -> AddQQ/1

== system ccu_form/Indication&Direction1 ==
  direction : Inport
  indication : Inport  Port=2
  Compare To Zero : simulink/Logic and Bit Operations/Compare To Zero  relop=>  OutDataTypeStr=boolean
  Compare To Zero1 : simulink/Logic and Bit Operations/Compare To Zero  relop=<  OutDataTypeStr=boolean
  GPIO_Write : GPIO_Lib/GPIO_Write  Port_name=GPIOB  Pin0=off  Toggle_Pin0=off  Pin1=off  Toggle_Pin1=off  Pin2=off  Toggle_Pin2=off  Pin3=off  Toggle_Pin3=off  Pin4=off  Toggle_Pin4=off  Pin5=off  Toggle_Pin5=off  Pin6=off  Toggle_Pin6=off  Pin7=off  Toggle_Pin7=off  Pin8=off  Toggle_Pin8=off  Pin9=off  Toggle_Pin9=off  Pin10=off  Toggle_Pin10=off  Pin11=off  Toggle_Pin11=off  Pin12=on  Toggle_Pin12=off  Pin13=on  Toggle_Pin13=off  Pin14=off  Toggle_Pin14=off  Pin15=off  Toggle_Pin15=off  PinList="GPIOB12  13  14  15GPIOC13"
      settings: SourceProductName=Target Support Package - STM32 Adapter
  GPIO_Write3 : GPIO_Lib/GPIO_Write  Port_name=GPIOC  Pin0=off  Toggle_Pin0=off  Pin1=off  Toggle_Pin1=off  Pin2=off  Toggle_Pin2=off  Pin3=off  Toggle_Pin3=off  Pin4=off  Toggle_Pin4=off  Pin5=off  Toggle_Pin5=off  Pin6=off  Toggle_Pin6=off  Pin7=off  Toggle_Pin7=off  Pin8=off  Toggle_Pin8=off  Pin9=off  Toggle_Pin9=off  Pin10=off  Toggle_Pin10=off  Pin11=off  Toggle_Pin11=off  Pin12=off  Toggle_Pin12=off  Pin13=on  Toggle_Pin13=off  Pin14=off  Toggle_Pin14=off  Pin15=off  Toggle_Pin15=off  PinList="GPIOB12  13  14  15GPIOC13"
      settings: SourceProductName=Target Support Package - STM32 Adapter
  Logical Operator1 : Logic  Operator=NOT  AllPortsSameDT=off  OutDataTypeStr=boolean
  wires:
  direction/1 -> Compare To Zero/1, Compare To Zero1/1
  Compare To Zero1/1 -> GPIO_Write/2
  Compare To Zero/1 -> GPIO_Write/1
  Logical Operator1/1 -> GPIO_Write3/1
  indication/1 -> Logical Operator1/1

== system ccu_form/Indication&Direction2 ==
  direction : Inport
  indication : Inport  Port=2
  Compare To Zero : simulink/Logic and Bit Operations/Compare To Zero  relop=>  OutDataTypeStr=boolean
  Compare To Zero1 : simulink/Logic and Bit Operations/Compare To Zero  relop=<  OutDataTypeStr=boolean
  GPIO_Write : GPIO_Lib/GPIO_Write  Port_name=GPIOB  Pin0=off  Toggle_Pin0=off  Pin1=off  Toggle_Pin1=off  Pin2=off  Toggle_Pin2=off  Pin3=off  Toggle_Pin3=off  Pin4=off  Toggle_Pin4=off  Pin5=off  Toggle_Pin5=off  Pin6=off  Toggle_Pin6=off  Pin7=off  Toggle_Pin7=off  Pin8=off  Toggle_Pin8=off  Pin9=off  Toggle_Pin9=off  Pin10=off  Toggle_Pin10=off  Pin11=off  Toggle_Pin11=off  Pin12=on  Toggle_Pin12=off  Pin13=on  Toggle_Pin13=off  Pin14=off  Toggle_Pin14=off  Pin15=off  Toggle_Pin15=off  PinList="GPIOB12  13  14  15GPIOC13"
      settings: SourceProductName=Target Support Package - STM32 Adapter
  GPIO_Write3 : GPIO_Lib/GPIO_Write  Port_name=GPIOC  Pin0=off  Toggle_Pin0=off  Pin1=off  Toggle_Pin1=off  Pin2=off  Toggle_Pin2=off  Pin3=off  Toggle_Pin3=off  Pin4=off  Toggle_Pin4=off  Pin5=off  Toggle_Pin5=off  Pin6=off  Toggle_Pin6=off  Pin7=off  Toggle_Pin7=off  Pin8=off  Toggle_Pin8=off  Pin9=off  Toggle_Pin9=off  Pin10=off  Toggle_Pin10=off  Pin11=off  Toggle_Pin11=off  Pin12=off  Toggle_Pin12=off  Pin13=on  Toggle_Pin13=off  Pin14=off  Toggle_Pin14=off  Pin15=off  Toggle_Pin15=off  PinList="GPIOB12  13  14  15GPIOC13"
      settings: SourceProductName=Target Support Package - STM32 Adapter
  Logical Operator1 : Logic  Operator=NOT  AllPortsSameDT=off  OutDataTypeStr=boolean
  wires:
  indication/1 -> Logical Operator1/1
  Logical Operator1/1 -> GPIO_Write3/1
  Compare To Zero/1 -> GPIO_Write/1
  Compare To Zero1/1 -> GPIO_Write/2
  direction/1 -> Compare To Zero1/1, Compare To Zero/1

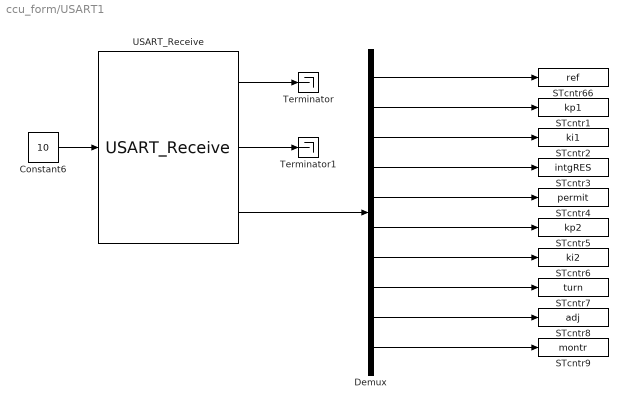
== system ccu_form/USART1 ==
  Constant6 : Constant  Value=10  OutDataTypeStr=uint8
  Demux : Demux  Outputs=10
  STcntr1 : DataStoreWrite  DataStoreName=kp1  DataStoreElements=kp1
  STcntr2 : DataStoreWrite  DataStoreName=ki1  DataStoreElements=ki1
  STcntr3 : DataStoreWrite  DataStoreName=intgRES  DataStoreElements=intgRES
  STcntr4 : DataStoreWrite  DataStoreName=permit  DataStoreElements=permit
  STcntr5 : DataStoreWrite  DataStoreName=kp2  DataStoreElements=kp2
  STcntr6 : DataStoreWrite  DataStoreName=ki2  DataStoreElements=ki2
  STcntr66 : DataStoreWrite  DataStoreName=ref  DataStoreElements=ref
  STcntr7 : DataStoreWrite  DataStoreName=turn  DataStoreElements=turn
  STcntr8 : DataStoreWrite  DataStoreName=adj  DataStoreElements=adj
  STcntr9 : DataStoreWrite  DataStoreName=montr  DataStoreElements=montr
  Terminator : Terminator
  Terminator1 : Terminator
  USART_Receive : USART_Lib/USART_Receive  USART_name=USART1  Buff_size=10  nbUsart=2  Soft_it=off  Soft_num=0  usartMode=Asynchronous  usartDma_Rx=off  usartDma_Tx=off  usartIt=on
      settings: SourceProductName=Target Support Package - STM32 Adapter
  wires:
  Demux/6 -> STcntr5/1
  Demux/4 -> STcntr3/1
  Demux/2 -> STcntr1/1
  Demux/7 -> STcntr6/1
  Demux/10 -> STcntr9/1
  Demux/5 -> STcntr4/1
  Demux/3 -> STcntr2/1
  Constant6/1 -> USART_Receive/1
  Demux/9 -> STcntr8/1
  Demux/8 -> STcntr7/1
  USART_Receive/3 -> Demux/1
  USART_Receive/2 -> Terminator1/1
  USART_Receive/1 -> Terminator/1
  Demux/1 -> STcntr66/1

== system ccu_form/Conversion from uint16 to float 1/Sign of reference ==
  Reference : Inport
  Delay2 : Delay  DelayLength=1  InitialCondition=0
  Gain7 : Gain  Gain=100  OutDataTypeStr=double
  Saturation4 : Saturate  UpperLimit=1  LowerLimit=-1
  Sign : Outport
  wires:
  Saturation4/1 -> Delay2/1
  Gain7/1 -> Saturation4/1
  Reference/1 -> Gain7/1
  Delay2/1 -> Sign/1

== system ccu_form/Conversion from uint16 to float 2/Sign of reference ==
  Reference : Inport
  Delay2 : Delay  DelayLength=1  InitialCondition=0
  Gain7 : Gain  Gain=100  OutDataTypeStr=double
  Saturation4 : Saturate  UpperLimit=1  LowerLimit=-1
  Sign : Outport
  wires:
  Delay2/1 -> Sign/1
  Reference/1 -> Gain7/1
  Gain7/1 -> Saturation4/1
  Saturation4/1 -> Delay2/1

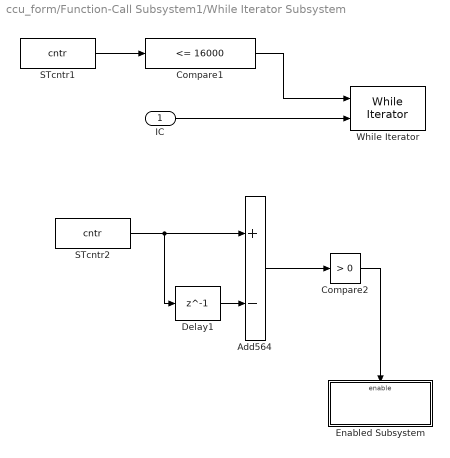
== system ccu_form/Function-Call Subsystem1/While Iterator Subsystem ==
  IC : Inport
  Add564 : Sum  Inputs=+-
  Compare1 : simulink/Logic and Bit Operations/Compare To Constant  relop=<=  const=16000  OutDataTypeStr=boolean
  Compare2 : simulink/Logic and Bit Operations/Compare To Constant  relop=>  const=0  OutDataTypeStr=boolean
  Delay1 : Delay  DelayLength=1  InitialCondition=0
  Enabled Subsystem : Subsystem  TreatAsAtomicUnit=on
  STcntr1 : DataStoreRead  DataStoreName=cntr  DataStoreElements=cntr
  STcntr2 : DataStoreRead  DataStoreName=cntr  DataStoreElements=cntr
  While Iterator : WhileIterator  MaxIters=1000000000
  wires:
  IC/1 -> While Iterator/2
  STcntr1/1 -> Compare1/1
  Compare1/1 -> While Iterator/1
  Delay1/1 -> Add564/2
  STcntr2/1 -> Delay1/1, Add564/1
  Add564/1 -> Compare2/1
  Compare2/1 -> Enabled Subsystem/Enable

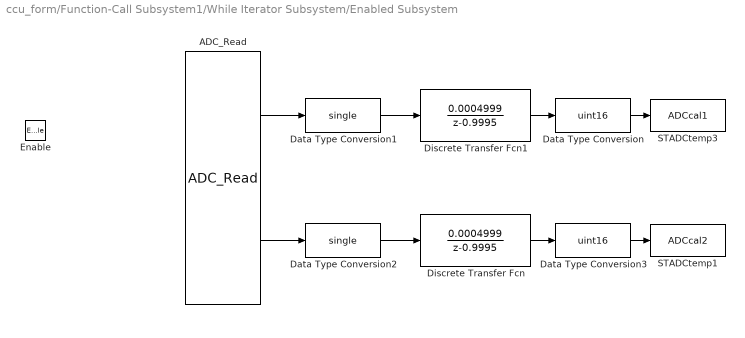
== system ccu_form/Function-Call Subsystem1/While Iterator Subsystem/Enabled Subsystem ==
  Enable : EnablePort
  ADC_Read : ADC_Lib/ADC_Read  ADC_Name=ADC1  ADC_Ch0=on  ADC_Ch1=on  ADC_Ch2=off  ADC_Ch3=off  ADC_Ch4=off  ADC_Ch5=on  ADC_Ch6=on  ADC_Ch7=off  ADC_Ch8=off  ADC_Ch9=off  ADC_Ch10=off  ADC_Ch11=off  ADC_Ch12=off  ADC_Ch13=off  ADC_Ch14=off  ADC_Ch15=off  ADC_Ch16=off  ADC_Ch17=off  ADC_Ch18=off  RgRk1=on  RgRk2=on  RgRk3=off  RgRk4=off  RgRk1_Ch=Ch0_r1  RgRk2_Ch=Ch1_r2  RgRk3_Ch=off  RgRk4_Ch=off  RgRk5=off  RgRk6=off  RgRk7=off  RgRk8=off  RgRk5_Ch=off  RgRk6_Ch=off  RgRk7_Ch=off  RgRk8_Ch=off  RgRk9=off  RgRk10=off  RgRk11=off  RgRk12=off  RgRk9_Ch=off  RgRk10_Ch=off  RgRk11_Ch=off  RgRk12_Ch=off  RgRk13=off  RgRk14=off  RgRk15=off  RgRk16=off  RgRk13_Ch=off  RgRk14_Ch=off  RgRk15_Ch=off  RgRk16_Ch=off  InjRk1=off  InjRk2=off  InjRk3=off  InjRk4=off  InjRk1_Ch=off  InjRk2_Ch=off  InjRk3_Ch=off  InjRk4_Ch=off  ADC_Trig=Not used  ADC_TrigEdge=Not used  DmaReq=off  DMA_Buffer=0  ItReq=off  AWD_Mode=NOT_USED  AWD_Ch=0  AWD_HThres=0  AWD_LThres=0  AWD_En_Int=off  AWD2_HThres=0  AWD2_LThres=0  AWD2_En_Int=off  AWD3_HThres=0  AWD3_LThres=0  AWD3_En_Int=off  EOC_SEQ=off  EOC_IT=off  JEOC_IT=off  AWD_IT=off  OVR_IT=off  CpltTrans=off  HalfTrans=off  ADC_RegNb=2  ADC_RegCh0=on  ADC_RegCh1=on  ADC_RegCh2=off  ADC_RegCh3=off  ADC_RegCh4=off  ADC_RegCh5=on  ADC_RegCh6=off  ADC_RegCh7=off  ADC_RegCh8=off  ADC_RegCh9=off  ADC_RegCh10=off  ADC_RegCh11=off  ADC_RegCh12=off  ADC_RegCh13=off  ADC_RegCh14=off  ADC_RegCh15=off  ADC_RegCh16=off  ADC_RegCh17=off  ADC_RegCh18=off  ADC_InjNb=2  ADC_InjCh0=off  ADC_InjCh1=on  ADC_InjCh2=off  ADC_InjCh3=off  ADC_InjCh4=off  ADC_InjCh5=on  ADC_InjCh6=on  ADC_InjCh7=off  ADC_InjCh8=off  ADC_InjCh9=off  ADC_InjCh10=off  ADC_InjCh11=off  ADC_InjCh12=off  ADC_InjCh13=off  ADC_InjCh14=off  ADC_InjCh15=off  ADC_InjCh16=off  ADC_InjCh17=off  ADC_InjCh18=off  ADC_RegRank0=1  ADC_RegRank1=2  ADC_RegRank2=0  ADC_RegRank3=0  ADC_RegRank4=0  ADC_RegRank5=2  ADC_RegRank6=0  ADC_RegRank7=0  ADC_RegRank8=0  ADC_RegRank9=0  ADC_RegRank10=0  ADC_RegRank11=0  ADC_RegRank12=0  ADC_RegRank13=0  ADC_RegRank14=0  ADC_RegRank15=0  ADC_RegRank16=0  ADC_RegRank17=0  ADC_RegRank18=0  ADC_InjRank0=0  ADC_InjRank1=0  ADC_InjRank2=0  ADC_InjRank3=0  ADC_InjRank4=0  ADC_InjRank5=0  ADC_InjRank6=0  ADC_InjRank7=0  ADC_InjRank8=0  ADC_InjRank9=0  ADC_InjRank10=0  ADC_InjRank11=0  ADC_InjRank12=0  ADC_InjRank13=0  ADC_InjRank14=0  ADC_InjRank15=0  ADC_InjRank16=0  ADC_InjRank17=0  ADC_InjRank18=0  NbADC=1  CurrentADC=ADC1
      settings: SourceProductName=Target Support Package - STM32 Adapter
  Data Type Conversion : DataTypeConversion  OutDataTypeStr=uint16
  Data Type Conversion1 : DataTypeConversion  OutDataTypeStr=single
  Data Type Conversion2 : DataTypeConversion  OutDataTypeStr=single
  Data Type Conversion3 : DataTypeConversion  OutDataTypeStr=uint16
  Discrete Transfer Fcn : DiscreteTransferFcn  Numerator=[0.0004999]  Denominator=[1 -0.9995]
  Discrete Transfer Fcn1 : DiscreteTransferFcn  Numerator=[0.0004999]  Denominator=[1 -0.9995]
  STADCtemp1 : DataStoreWrite  DataStoreName=ADCcal2  DataStoreElements=ADCcal2
  STADCtemp3 : DataStoreWrite  DataStoreName=ADCcal1  DataStoreElements=ADCcal1
  wires:
  Discrete Transfer Fcn1/1 -> Data Type Conversion/1
  Data Type Conversion/1 -> STADCtemp3/1
  Data Type Conversion1/1 -> Discrete Transfer Fcn1/1
  ADC_Read/1 -> Data Type Conversion1/1
  ADC_Read/2 -> Data Type Conversion2/1
  Data Type Conversion2/1 -> Discrete Transfer Fcn/1
  Discrete Transfer Fcn/1 -> Data Type Conversion3/1
  Data Type Conversion3/1 -> STADCtemp1/1
